simulink model "PressuredropFittingSimulation"  (R2022a)
settings: Solver=VariableStepAuto  StartTime=0.0  StopTime=10.0  RelTol=1e-3
settings Model: Creator=StephenDennis  LastModifiedBy=StephenDennis

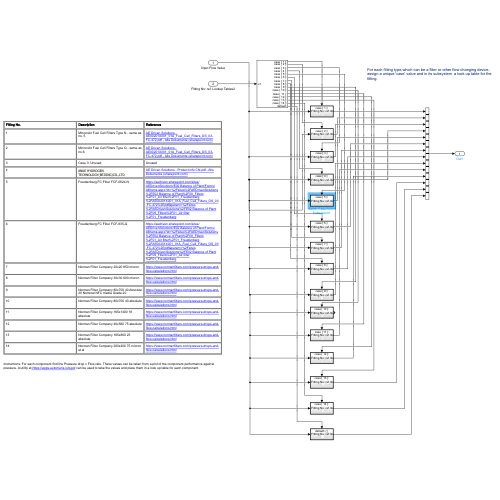
[thumbnail: Simulink's stored preview of the top-level diagram]
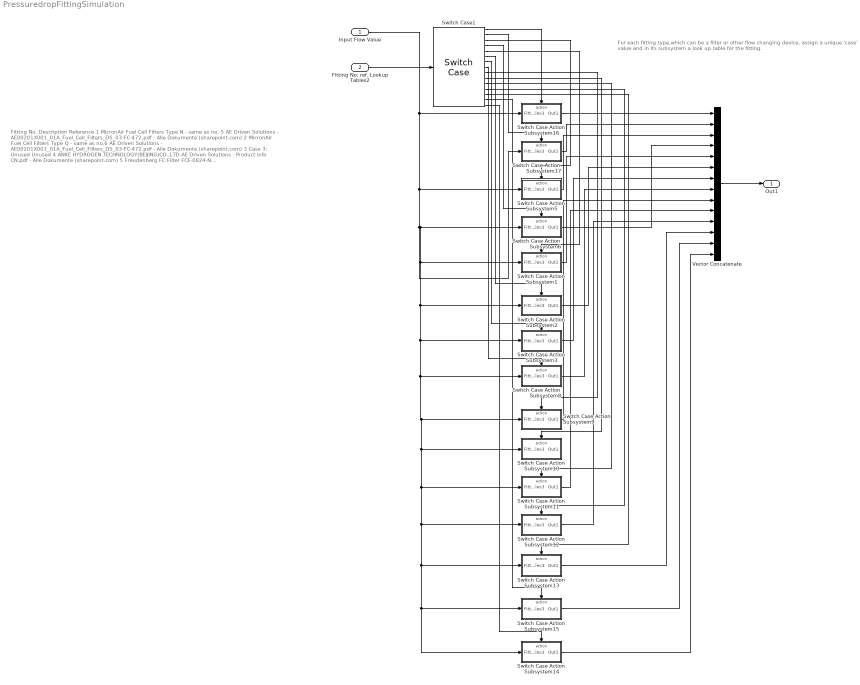
== system PressuredropFittingSimulation ==
  note: Fitting No.
      | Description
      | Reference
      |
      | 1
      | MicronAir Fuel Cell Filters Type N - same as no. 5
      | AE Driven Solutions - AE00201X001_01A_Fuel_Cell_Filters_DS_03-FC-472.pdf - Alle Dokumente (sharepoint.com)
      |
      | 2
      | MicronAir Fuel Cell Filters Type Q - same as no.6
      | AE Driven Solutions - AE00201X001_01A_Fuel_Cell_Filters_DS_03-FC-472.pdf - Alle Dokumente (sharepoint.com)
      |
      | 3
      | Case 3: Unused
      | Unused
      |
      | 4
      | ANKE HYDROGEN TECHNOLOGY(BEIJING)CO.,LTD
      | AE Driven Solutions - Product info CN.pdf - Alle Dokumente (sharepoint.com)
      |
      | 5
      | Freudenberg FC Filter FCF-0824-N
      | https://aedriven.sharepoint.com/sites/AEDrivenSolutions/E02 Balance of Plant/Forms/AllItems.aspx?id=%2Fsites%2FAEDrivenSolutions%2FE02 Balance of Plant%2F09_Filters%2F01_Air filter%2F01_Freudenberg%2FAE00201X001_01A_Fuel_Cell_Filters_DS_03-FC-472%2Epdf&parent=%2Fsites%2FAEDrivenSolutions%2FE02 Balance of Plant%2F09_Filters%2F01_Air filter%2F01_Freudenberg
      |
      | 6
      | Freudenberg FC Filter FCF-835-Q
      | https://aedriven.sharepoint.com/sites/AEDrivenSolutions/E02 Balance of Plant/Forms/AllItems.aspx?id=%2Fsites%2FAEDrivenSolutions%2FE02 Balance of Plant%2F09_Filters%2F01_Air filter%2F01_Freudenberg%2FAE00201X001_01A_Fuel_Cell_Filters_DS_03-FC-472%2Epdf&parent=%2Fsites%2FAEDrivenSolutions%2FE02 Balance of Plant%2F09_Filters%2F01_Air filter%2F01_Freudenberg
      |
      | 7
      | Norman Filter Company 20x20 850 micron
      | https://www.normanfilters.com/pressure-drops-and-flow-calculations.html
      |
      | 8
      | Norman Filter Company 30x30 600 micron
      | https://www.normanfilters.com/pressure-drops-and-flow-calculations.html
      |
      | 9
      | Norman Filter Company 80x700 40 Absolute 20 Nominal NFC media Grade 20
      | https://www.normanfilters.com/pressure-drops-and-flow-calculations.html
      |
      | 10
      | Norman Filter Company 80x700 40 absolute
      | https://www.normanfilters.com/pressure-drops-and-flow-calculations.html
      |
      | 11
      | Norman Filter Company 165x1400 18 absolute
      | https://www.normanfilters.com/pressure-drops-and-flow-calculations.html
      |
      | 12
      | Norman Filter Company 40x560 75 absolute
      | https://www.normanfilters.com/pressure-drops-and-flow-calculations.html
      |
      | 13
      | Norman Filter Company 165x800 25 absolute
      | https://www.normanfilters.com/pressure-drops-and-flow-calculations.html
      |
      | 14
      | Norman Filter Company 200x200 75 micron et al
      | https://www.normanfilters.com/pressure-drops-and-flow-calculations.html
      |
      | Instructions: For each component find the Pressure drop v Flow rate. These values can be taken from a plot of the component performance against
      | pressure. A utility at https://apps.automeris.io/wpd/ can be used to take the values and place them in a look up table for each component.
  note: For each fitting type,which can be a filter or other flow changing device, assign a unique 'case' value and in its subsystem a look up table for the fitting.
  Input Flow Value : Inport
  Fitting No: ref. Lookup Tables2 : Inport  Port=2
  Switch Case Action Subsystem1 : Subsystem  TreatAsAtomicUnit=on
  Switch Case Action Subsystem10 : Subsystem  TreatAsAtomicUnit=on
  Switch Case Action Subsystem11 : Subsystem  TreatAsAtomicUnit=on
  Switch Case Action Subsystem12 : Subsystem  TreatAsAtomicUnit=on
  Switch Case Action Subsystem13 : Subsystem  TreatAsAtomicUnit=on
  Switch Case Action Subsystem14 : Subsystem  TreatAsAtomicUnit=on
  Switch Case Action Subsystem15 : Subsystem  TreatAsAtomicUnit=on
  Switch Case Action Subsystem16 : Subsystem  TreatAsAtomicUnit=on
  Switch Case Action Subsystem17 : Subsystem  TreatAsAtomicUnit=on
  Switch Case Action Subsystem2 : Subsystem  TreatAsAtomicUnit=on
  Switch Case Action Subsystem3 : Subsystem  TreatAsAtomicUnit=on
  Switch Case Action Subsystem5 : Subsystem  TreatAsAtomicUnit=on
  Switch Case Action Subsystem6 : Subsystem  TreatAsAtomicUnit=on
  Switch Case Action Subsystem8 : Subsystem  TreatAsAtomicUnit=on
  Switch Case Action Subsystem9 : Subsystem  TreatAsAtomicUnit=on
  Switch Case1 : SwitchCase  CaseConditions={1,2,3,4,5,6,7,8,9,10,11,12,13,14}
  Vector Concatenate : Concatenate  NumInputs=14
  Out1 : Outport
  wires:
  Switch Case1/15 -> Switch Case Action Subsystem14/Action
  Switch Case Action Subsystem16/1(Out1) -> Vector Concatenate/1
  Switch Case1/2 -> Switch Case Action Subsystem17/Action
  Switch Case1/1 -> Switch Case Action Subsystem16/Action
  Vector Concatenate/1 -> Out1/1
  Switch Case Action Subsystem6/1(Out1) -> Vector Concatenate/4
  Fitting No: ref. Lookup Tables2/1 -> Switch Case1/1
  Switch Case Action Subsystem5/1(Out1) -> Vector Concatenate/3
  Switch Case1/3 -> Switch Case Action Subsystem5/Action
  Switch Case Action Subsystem17/1(Out1) -> Vector Concatenate/2
  Input Flow Value/1 -> Switch Case Action Subsystem17/1(Fitting No: ref. Lookup Tables3), Switch Case Action Subsystem15/1(Fitting No: ref. Lookup Tables3), Switch Case Action Subsystem14/1(Fitting No: ref. Lookup Tables3), Switch Case Action Subsystem13/1(Fitting No: ref. Lookup Tables3), Switch Case Action Subsystem12/1(Fitting No: ref. Lookup Tables3), Switch Case Action Subsystem11/1(Fitting No: ref. Lookup Tables3), Switch Case Action Subsystem10/1(Fitting No: ref. Lookup Tables3), Switch Case Action Subsystem9/1(Fitting No: ref. Lookup Tables3), Switch Case Action Subsystem8/1(Fitting No: ref. Lookup Tables3), Switch Case Action Subsystem3/1(Fitting No: ref. Lookup Tables3), Switch Case Action Subsystem2/1(Fitting No: ref. Lookup Tables3), Switch Case Action Subsystem1/1(Fitting No: ref. Lookup Tables3), Switch Case Action Subsystem6/1(Fitting No: ref. Lookup Tables3), Switch Case Action Subsystem5/1(Fitting No: ref. Lookup Tables3), Switch Case Action Subsystem16/1(Fitting No: ref. Lookup Tables3)
  Switch Case1/4 -> Switch Case Action Subsystem6/Action
  Switch Case1/5 -> Switch Case Action Subsystem1/Action
  Switch Case1/6 -> Switch Case Action Subsystem2/Action
  Switch Case Action Subsystem1/1(Out1) -> Vector Concatenate/5
  Switch Case Action Subsystem2/1(Out1) -> Vector Concatenate/6
  Switch Case1/7 -> Switch Case Action Subsystem3/Action
  Switch Case1/8 -> Switch Case Action Subsystem8/Action
  Switch Case1/9 -> Switch Case Action Subsystem9/Action
  Switch Case1/10 -> Switch Case Action Subsystem10/Action
  Switch Case1/11 -> Switch Case Action Subsystem11/Action
  Switch Case1/12 -> Switch Case Action Subsystem12/Action
  Switch Case1/13 -> Switch Case Action Subsystem13/Action
  Switch Case Action Subsystem3/1(Out1) -> Vector Concatenate/7
  Switch Case Action Subsystem8/1(Out1) -> Vector Concatenate/8
  Switch Case Action Subsystem9/1(Out1) -> Vector Concatenate/9
  Switch Case Action Subsystem11/1(Out1) -> Vector Concatenate/10
  Switch Case Action Subsystem12/1(Out1) -> Vector Concatenate/11
  Switch Case Action Subsystem13/1(Out1) -> Vector Concatenate/12
  Switch Case Action Subsystem14/1(Out1) -> Vector Concatenate/14
  Switch Case Action Subsystem15/1(Out1) -> Vector Concatenate/13
  Switch Case1/14 -> Switch Case Action Subsystem15/Action

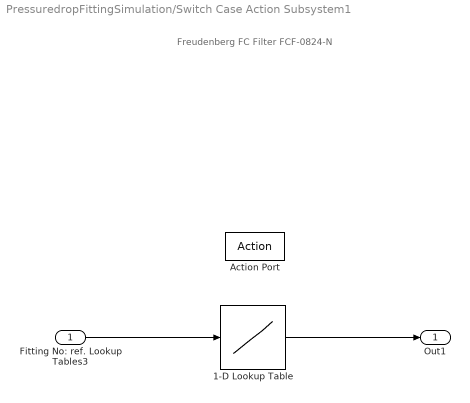
== system PressuredropFittingSimulation/Switch Case Action Subsystem1 ==
  note: Freudenberg FC Filter FCF-0824-N
  Fitting No: ref. Lookup Tables3 : Inport
  Action Port : ActionPort  ActionPortLabel=case [ 5 ]:
  1-D Lookup Table : Lookup_n-D  NumberOfTableDimensions=1  BreakpointsForDimension1=[0.225255973;4.325938567;10.54607509;16.30546075;21.37372014;28.05460751;33.29564846;38.70947099;44.00170648;50.70819113;55.99585568;61.59068747;66.98805461;72.05631399;77.12457338;82.19283276;87.26109215;92.32935154;97.39761092;102.4658703;107.5341297;112.6023891;117.6706485;122.7389078;127.8071672;132.8754266;137.943686;143.0119454;148.0802048;153.1484642;158.2167235;163.2849829;168.3532423;173.4215017;178.4897611;183.5580205;188.6262799;193.6945392;198.7627986;203.831058;208.8993174;213.9675768;219.0358362;224.1040956;229.1723549;234.2406143;239.3088737;244.3771331;249.4453925;254.5136519;259.5819113;264.6501706;269.71843;274.7866894;279.8549488;284.9232082;289.9914676;295.059727;300.1279863]  Table=[2.196382429;4.992617202;0.839793282;2.777777778;8.06319004;6.65374677;9.318475452;11.25645995;16.12833764;19.57364341;25.7567368;30.74012551;26.82640357;29.82147052;33.4331689;36.78059666;40.30420484;44.62062485;48.67277425;52.30209067;54.92717876;58.97932817;63.38383838;67.96452901;74.39511393;80.20906742;86.99201315;94.65586093;103.1125206;112.802443;123.0209067;133.9440921;145.3077284;157.3760864;170.0610759;182.7460653;196.2238666;209.7016678;223.3556495;237.5381724;252.0730561;265.815128;280.2619215;294.5325346;309.2435988;324.3070237;338.9299977;353.9053324;369.1449377;384.7369039;399.9765093;416.1851069;432.9222457;450.0117454;466.7488842;484.0145642;501.2802443;519.0744656;536.6925065]  InternalRulePriority=Speed  RndMeth=Simplest
  Out1 : Outport
  wires:
  Fitting No: ref. Lookup Tables3/1 -> 1-D Lookup Table/1
  1-D Lookup Table/1 -> Out1/1

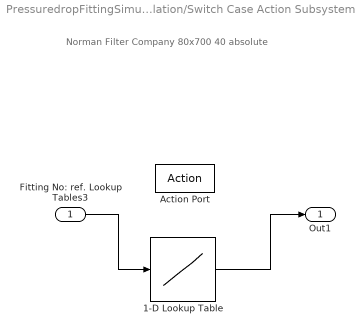
== system PressuredropFittingSimulation/Switch Case Action Subsystem10 ==
  note: Norman Filter Company 80x700 40 absolute
  Fitting No: ref. Lookup Tables3 : Inport
  Action Port : ActionPort  ActionPortLabel=case [ 10 ]:
  1-D Lookup Table : Lookup_n-D  NumberOfTableDimensions=1  BreakpointsForDimension1="[5.731513805\t36.87083466\t68.01015551\t99.14947636\t130.2887972\t161.4281181\t192.5674389\t223.7067598\t254.8460806\t285.9854015\t319.5511629\t347.1752557\t379.403364\t410.5426849\t441.6820057\t472.8213266\t505.9204648\t532.6021618\t566.2392891\t597.37861\t628.9897387\t661.4770821\t692.5844761\t723.2569555\t754.3490955\t782.9760394\t815.9498238\t847.3778166\t878.4817518\t908.0978072\t940.9019359\t969.2625566\t1001.088896\t1033.059497\t1064.021447\t1095.607744\t1126.747064\t1157.886385\t1188.08209\t1218.666343\t1252.578229\t1282.443669\t1313.58299\t1344.72231\t1375.861631\t1404.503146\t1438.140273\t1469.279594\t1500.418915\t1531.558235\t1562.697556\t1593.836877\t1624.302187\t1653.958683\t1684.423992\t1715.563313\t1746.702634\t1777.841955\t1808.981276\t1840.120597\t1871.259917\t1902.399238\t1933.538559\t1964.67788\t1991.975337]"  Table="[0.699801063\t0.441503285\t0.567587624\t0.66857184\t0.739494281\t0.924117777\t1.251420046\t1.487828181\t1.74174803\t2.153273303\t2.335270042\t2.787736162\t3.44914012\t4.070805958\t4.674960082\t5.121508782\t5.432678465\t5.614412019\t6.723830589\t7.389275711\t8.046613559\t8.717083537\t9.404423003\t10.15898256\t10.99651675\t11.97860858\t12.78445989\t13.65971572\t14.42213804\t14.9686396\t15.97143584\t16.60239751\t17.58855759\t18.48668233\t19.51709572\t20.69793494\t21.81114485\t22.93967751\t24.12755543\t25.37020037\t26.92709473\t28.21070335\t29.51970395\t30.63169777\t32.01074523\t33.25665216\t34.3310473\t35.67944926\t37.04536293\t38.73524331\t40.09677905\t41.53273958\t43.32623092\t45.24793303\t46.96137083\t48.55931471\t50.04343245\t51.74206869\t53.07733686\t54.66214695\t56.3170039\t58.31333927\t60.23087192\t62.32352171\t63.53620789]"  InternalRulePriority=Speed  RndMeth=Simplest
  Out1 : Outport
  wires:
  Fitting No: ref. Lookup Tables3/1 -> 1-D Lookup Table/1
  1-D Lookup Table/1 -> Out1/1

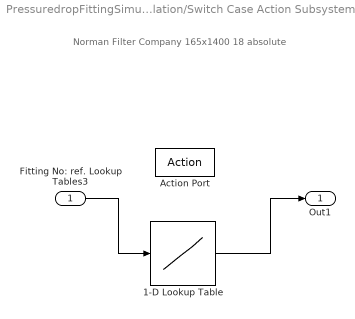
== system PressuredropFittingSimulation/Switch Case Action Subsystem11 ==
  note: Norman Filter Company 165x1400 18 absolute
  Fitting No: ref. Lookup Tables3 : Inport
  Action Port : ActionPort  ActionPortLabel=case [ 11 ]:
  1-D Lookup Table : Lookup_n-D  NumberOfTableDimensions=1  BreakpointsForDimension1=[19.50347696 50.62498646 81.74649596 112.8680055 143.989515 175.1110245 206.232534 237.3540435 268.475553 299.5970625 330.718572 361.8400815 392.961591 424.0831005 455.20461 486.3261195 517.447629 548.5691385 579.6906479 610.8121574 641.9336669 673.0551764 704.1766859 735.2981954 766.4197049 797.5412144 828.6627239 859.7842334 890.9057429 922.0272524 953.1487619 984.2702714 1015.391781 1046.51329 1077.6348 1108.756309 1139.877819 1170.999328 1202.120838 1233.242347 1264.363857 1295.485366 1326.606876 1357.728385 1388.849895 1419.971404 1451.092914 1482.214423 1513.335933 1544.457442 1575.578952 1606.700461 1637.821971 1668.94348 1700.06499 1731.186499 1762.308009 1793.429518 1824.551028 1855.672537 1886.794047 1917.915556 1949.037066 1980.158575 1998.548558]  Table=[0.0953884904119775 0.5159225300020438 1.0021650132780877 1.4066369888560644 1.7746042734973884 2.0023935449420236 2.3440774521089764 2.677000233451139 3.088773147216429 3.491784935156943 3.921080100571814 4.4423670871470335 5.071707958894706 5.529622802003914 5.8835722853255845 6.453045463937173 7.031279768373551 7.565708443685949 8.152703873947118 8.774743807507463 9.53696175426451 10.167762813649645 10.894936257107517 11.429364932419915 12.165299501702592 12.980084203408381 13.707257646866267 14.42566996449932 15.152843407957207 16.12532837450928 16.817457314667976 17.535869632301058 18.4207433406052 19.28809479725976 20.17880925611375 21.110408968816827 21.995282677120997 22.915200888724314 23.931491484400368 24.87769307347807 25.87646141750453 26.936557642304564 28.057981747878145 29.100555721028584 30.1518908200038 31.2557926739278 32.342172276202206 33.48111863342538 34.646348368122915 35.84662260611964 37.04689684411636 38.17708207551473 39.39487856516105 40.621436180632145 41.90056055105201 43.16216266982228 44.41500366276776 45.78173929143557 47.1046692909794 48.445121542172814 49.79433491919103 51.17859279950841 52.57161180565059 53.9295863084936 54.38516485138287]  InternalRulePriority=Speed  RndMeth=Simplest
  Out1 : Outport
  wires:
  Fitting No: ref. Lookup Tables3/1 -> 1-D Lookup Table/1
  1-D Lookup Table/1 -> Out1/1

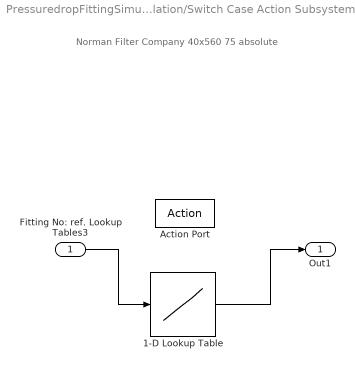
== system PressuredropFittingSimulation/Switch Case Action Subsystem12 ==
  note: Norman Filter Company 40x560 75 absolute
  Fitting No: ref. Lookup Tables3 : Inport
  Action Port : ActionPort  ActionPortLabel=case [ 12 ]:
  1-D Lookup Table : Lookup_n-D  NumberOfTableDimensions=1  BreakpointsForDimension1="[93.06340850501508 124.18491800437602 155.30642750373698 186.4279370030979 217.5494465024588 248.67095600181977 279.7924655011807 310.91397500054165 339.20625636359705 381.6446784081802 421.25387231645766 460.86306622473523 499.05764606486 538.6668399731376 576.8614198132624 615.0559996533872 656.0798076298175 694.2743874699423 731.0543532419143 772.0781612183447 808.8581269903167 848.4673208985943 888.0765148068717 924.8564805788437 964.4656744871213 1002.6602543272461 1040.8548341673709 1079.0494140074957 1117.2439938476205 1155.4385736877452 1192.2185394597172  1231.8277333679948 1268.6076991399668 1306.8022789800916 1343.5822447520636 1378.9475964558828 1415.727562227855 1453.9221420679798 1492.1167219081044 1527.4820736119239 1565.6766534520486 1602.4566192240206 1639.2365849959926 1677.4311648361174 1712.7965165399366 1749.5764823119086 1786.3564480838807 1823.1364138558527 1857.087151491519 1895.2817313316439 1930.6470830354633 1967.4270488074353 1994.3047161023378]"  Table="[0.039901360188252966 0.1450348700857944 0.19760162503455092 0.30273513493206394 0.31149626075686854 0.3377796382312539 0.504241028902328 0.7419595762817295 1.2090249285857055 1.7520756642336437 2.041192816451826  2.426682352742745 2.8379859204817137 3.2756771648120377 3.6795233456882244 4.143028621466598 4.670782153293445 5.219186910278722 5.684986766630274  6.254042748774012 6.763439636015576 7.396743874207772 8.08511804615587 8.71842228434808 9.406796456296135 10.102054369963696 10.811079767070211 11.531578067042503 12.339270428794919 13.121722404242547 13.94088766886074 14.840363253539564 15.643466454145639 16.593422811433967 17.551639658785675 18.390079400218426 19.353803240945723 20.324410823392498 21.36156124246091 22.320695922041878 23.401443372000358 24.461539596800378 25.54572891761859 26.712523139070555 27.770324783297426 28.926793392170183 30.099324065055043 31.30397886596417 32.460447474836926 33.72292570618967 34.95006739671577 36.202908389661246 37.23088048643703]"  InternalRulePriority=Speed  RndMeth=Simplest
  Out1 : Outport
  wires:
  Fitting No: ref. Lookup Tables3/1 -> 1-D Lookup Table/1
  1-D Lookup Table/1 -> Out1/1

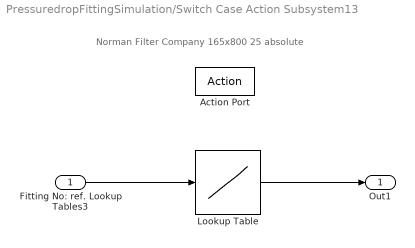
== system PressuredropFittingSimulation/Switch Case Action Subsystem13 ==
  note: Norman Filter Company 165x800 25 absolute
  Fitting No: ref. Lookup Tables3 : Inport
  Action Port : ActionPort  ActionPortLabel=case [ 13 ]:
  " Lookup Table" : Lookup_n-D  NumberOfTableDimensions=1  BreakpointsForDimension1="[11.015792552154437 42.13730205151538 73.25881155087632 104.38032105023723 135.5018305495982 166.6233400489591 197.74484954832008 228.866359047681 259.98786854704196 291.10937804640287 322.23088754576384 353.35239704512475 384.47390654448566 415.5954160438466 446.7169255432076 477.83843504256845 508.9599445419294 540.0814540412904  571.2029635406514 602.3244730400122 633.1630597257425 663.435800784212 695.6890015380951 726.810511037456 757.9320205368169 788.1104539907427 820.1750395355389 851.2965490348997 882.4180585342607 913.5395680336217 944.6610775329825 974.3679729641908 1006.9040965317045 1038.0256060310653 1069.1471155304264 1099.7027794025262 1129.9755204609955 1162.5116440285092 1193.63315352787  1224.7546630272311 1255.876172526592 1286.9976820259528 1318.119191525314 1349.2407010246748 1380.3622105240356 1411.4837200233967 1442.6052295227576 1473.7267390221184 1504.8482485214795 1535.9697580208403 1567.0912675202014 1598.2127770195623 1629.3342865189231 1660.4557960182842 1692.1431511449064 1722.698815017006 1752.2485311073083 1784.9418340157279 1816.063343515089 1847.1848530144498 1878.3063625138107 1909.4278720131717 1940.5493815125324 1971.6708910118937 1992.4185640114674]"  Table=[-0.07224105036908668 -0.15284340795720652 -0.222932414555558 -0.31930479862828065 -0.345588176102666 -0.24921579202991495 -0.03310802168498128 -0.2170916640056788 -0.24921579202992916 -0.17036565960677308 0.2676906316329024 0.99486407509076 1.0561919558643211 1.4329203663304355 2.2418643174863604 2.536822220254436 2.457972087831294 2.5280610944296456 2.4930165911304556 2.708540286420387 3.066870332654446 3.346350246465363 3.3603680477850304 3.8509910939734766 4.122585994542078 4.185860792165585 4.534358908307368 4.97241519954704 5.3929492391371525 5.734633146304091 6.1639283117189905 6.574825112901806 6.908624006826415 7.092607649147098 7.250307913993396 7.760205436996372 8.174606688509101 8.581999039362003 8.967488575652922 9.352978111943841 9.791034403183517 10.264135197722382 10.632102482363706 10.912458508757112 11.574799621111495 11.884943475309186 12.366805395672827 12.874950693510854 13.234156852327402 13.963082520950195 14.332802030756525 14.802398374965449 15.310543672803476 16.05523936791093 16.414445526727476 17.0036020346920 17.26038089803255 17.76365890374568 18.324370956532462 18.928888638443226 19.623937953876847 20.181729631388706 20.558458041854834 21.040319962218476 21.350853199786187]  InternalRulePriority=Speed  RndMeth=Simplest
  Out1 : Outport
  wires:
  Fitting No: ref. Lookup Tables3/1 -> " Lookup Table"/1
  " Lookup Table"/1 -> Out1/1

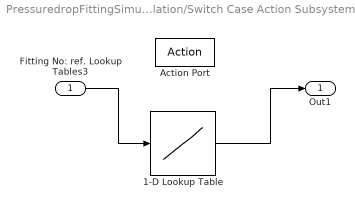
== system PressuredropFittingSimulation/Switch Case Action Subsystem14 ==
  Fitting No: ref. Lookup Tables3 : Inport
  Action Port : ActionPort  ActionPortLabel=default:
  1-D Lookup Table : Lookup_n-D  NumberOfTableDimensions=1  BreakpointsForDimension1=0  Table=0  InternalRulePriority=Speed  RndMeth=Simplest
  Out1 : Outport
  wires:
  Fitting No: ref. Lookup Tables3/1 -> 1-D Lookup Table/1
  1-D Lookup Table/1 -> Out1/1

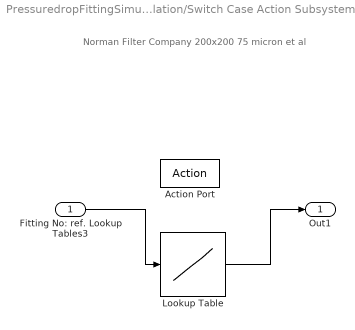
== system PressuredropFittingSimulation/Switch Case Action Subsystem15 ==
  note: Norman Filter Company 200x200 75 micron et al
  Fitting No: ref. Lookup Tables3 : Inport
  Action Port : ActionPort  ActionPortLabel=case [ 14 ]:
  " Lookup Table" : Lookup_n-D  NumberOfTableDimensions=1  BreakpointsForDimension1=|  Table=|  InternalRulePriority=Speed  RndMeth=Simplest
      BreakpointsForDimension1=|
      | [31.16364558	62.25757384	93.35150209	124.4454303	155.5393586	186.6332869	217.7272151	248.8211434	279.9150716	311.0089999	342.1029281	373.1968564	404.2907846	435.3847129	466.4786411	497.5725694	528.6664977	559.7604259	591.9415545	621.9482824	653.0422107	684.1361389	715.2300672	746.3239954	777.4179237	808.5118519	839.6057802	870.6997085	902.0291968	932.887565	963.9814932	995.7277416	1024.755989	1054.436557	1085.530485	1116.624414	1146.304982	1175.985549	1205.992277	1238.173406	1265.498373	1297.534542	1326.272869	1354.540077	1382.336164	1410.603372	1438.022563	1467.137787	1496.175918	1521.451207	1550.911511	1579.178718	1603.591307	1626.847509	1653.701356	1679.141843	1704.58233	1729.765842	1754.049943	1780.19711	1806.874287	1837.873085	1863.649616	1893.26594	1913.557757	1937.786792	1959.639518	1984.427684	2002.801369
      | ]
      Table=|
      | [-22.67333548	-21.7831509	-20.81586371	-19.69086666	-18.63946754	-17.44087255	-16.14765164	-15.0121406	-13.80303161	-12.43621276	-11.05887992	-9.702575063	-8.20958832	-6.895339426	-5.602118514	-3.804226027	-2.132501434	-0.45026285	1.230762582	2.987812257	4.75416277	6.383831399	8.339433753	10.04270032	12.09292859	14.08007292	16.14081519	18.42235127	20.33214961	22.64360189	24.55200811	26.82042417	29.17185582	31.30199043	33.37324669	35.75992268	38.06564094	40.45967672	42.72827251	45.29611265	47.63021869	50.3533424	52.80465996	55.56643232	58.09047166	60.74326845	63.02606621	65.57760158	67.96427758	70.57489741	73.33692705	75.93388287	78.19439097	80.79975797	83.41867635	85.98876307	88.57170023	91.06351614	93.84840954	96.02173913	99.13415431	102.2873634	105.1102083	107.6353185	110.0420212	112.7433659	115.3411305	118.3473232	119.4512922
      | ]
  Out1 : Outport
  wires:
  Fitting No: ref. Lookup Tables3/1 -> " Lookup Table"/1
  " Lookup Table"/1 -> Out1/1

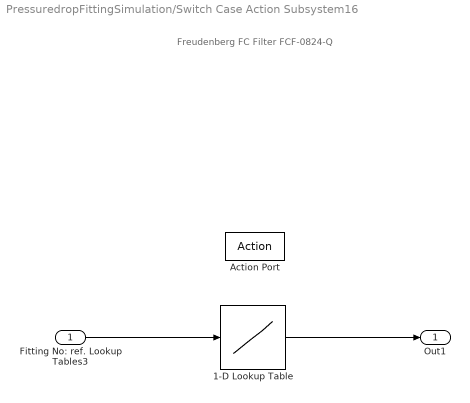
== system PressuredropFittingSimulation/Switch Case Action Subsystem16 ==
  note: Freudenberg FC Filter FCF-0824-Q
  Fitting No: ref. Lookup Tables3 : Inport
  Action Port : ActionPort  ActionPortLabel=case [ 1 ]:
  1-D Lookup Table : Lookup_n-D  NumberOfTableDimensions=1  BreakpointsForDimension1=[0.225255973;4.325938567;10.54607509;16.30546075;21.37372014;28.05460751;33.29564846;38.70947099;44.00170648;50.70819113;55.99585568;61.59068747;66.98805461;72.05631399;77.12457338;82.19283276;87.26109215;92.32935154;97.39761092;102.4658703;107.5341297;112.6023891;117.6706485;122.7389078;127.8071672;132.8754266;137.943686;143.0119454;148.0802048;153.1484642;158.2167235;163.2849829;168.3532423;173.4215017;178.4897611;183.5580205;188.6262799;193.6945392;198.7627986;203.831058;208.8993174;213.9675768;219.0358362;224.1040956;229.1723549;234.2406143;239.3088737;244.3771331;249.4453925;254.5136519;259.5819113;264.6501706;269.71843;274.7866894;279.8549488;284.9232082;289.9914676;295.059727;300.1279863]  Table=[2.196382429;4.992617202;0.839793282;2.777777778;8.06319004;6.65374677;9.318475452;11.25645995;16.12833764;19.57364341;25.7567368;30.74012551;26.82640357;29.82147052;33.4331689;36.78059666;40.30420484;44.62062485;48.67277425;52.30209067;54.92717876;58.97932817;63.38383838;67.96452901;74.39511393;80.20906742;86.99201315;94.65586093;103.1125206;112.802443;123.0209067;133.9440921;145.3077284;157.3760864;170.0610759;182.7460653;196.2238666;209.7016678;223.3556495;237.5381724;252.0730561;265.815128;280.2619215;294.5325346;309.2435988;324.3070237;338.9299977;353.9053324;369.1449377;384.7369039;399.9765093;416.1851069;432.9222457;450.0117454;466.7488842;484.0145642;501.2802443;519.0744656;536.6925065]  InternalRulePriority=Speed  RndMeth=Simplest
  Out1 : Outport
  wires:
  Fitting No: ref. Lookup Tables3/1 -> 1-D Lookup Table/1
  1-D Lookup Table/1 -> Out1/1

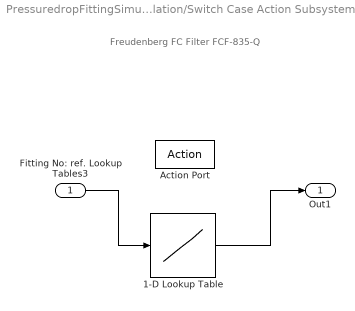
== system PressuredropFittingSimulation/Switch Case Action Subsystem17 ==
  note: Freudenberg FC Filter FCF-835-Q
  Fitting No: ref. Lookup Tables3 : Inport
  Action Port : ActionPort  ActionPortLabel=case [ 2 ]:
  1-D Lookup Table : Lookup_n-D  NumberOfTableDimensions=1  BreakpointsForDimension1=|  Table="[0.743908154\t3.467666354\t7.070056232\t7.860824742\t7.860824742\t7.94868791\t11.19962512\t12.78116214\t17.87722587\t19.45876289\t19.02920962\t22.00679475\t26.31208997\t32.11105904\t35.97703843\t38.61293346\t42.12746017\t46.60848172\t50.91377694\t56.09770384\t60.8423149\t65.58692596\t71.38589503\t78.15135895\t86.76194939\t96.33903468\t105.6525305\t114.7024367\t124.5431115\t134.4716495\t144.5759138\t154.9437676\t166.7174321\t177.7881912\t190.0011715\t203.7078257\t217.0630272\t229.8910497\t242.5433458\t255.8106842\t269.868791\t283.8390347\t297.8971415\t311.6916589\t325.1347235\t340.071462\t355.5353796\t370.3842549\t385.8481724\t401.3999531\t416.0731022\t432.239925\t448.6703374\t465.7377577\t482.0583411\t498.6644799\t517.3109966\t532.9311153\t550.5037488\t566.0806333]"  InternalRulePriority=Speed  RndMeth=Simplest
      | [1.454081633	6.505102041	11.55612245	16.60714286	21.65816327	26.70918367	31.76020408	36.81122449	41.8622449	46.91326531	51.50510204	57.4744898	62.5255102	67.57653061	72.62755102	77.67857143	82.72959184	87.78061224	92.83163265	97.88265306	102.9336735	107.9846939	113.0357143	118.0867347	123.1377551	128.1887755	133.2397959	138.2908163	143.3418367	148.3928571	153.4438776	158.494898	163.5459184	168.5969388	173.6479592	178.6989796	183.75	188.8010204	193.8520408	198.9030612	203.9540816	209.005102	214.0561224	219.1071429	224.1581633	229.2091837	234.2602041	239.3112245	244.3622449	249.4132653	254.4642857	259.5153061	264.5663265	269.3877551	274.6683673	279.7193878	285.0255102	289.8214286	294.872449	299.005102
      | ]
  Out1 : Outport
  wires:
  Fitting No: ref. Lookup Tables3/1 -> 1-D Lookup Table/1
  1-D Lookup Table/1 -> Out1/1

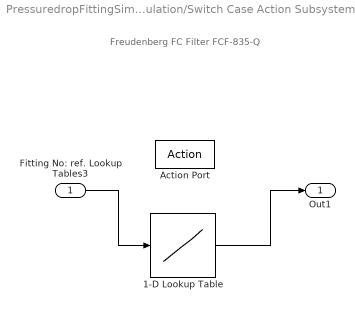
== system PressuredropFittingSimulation/Switch Case Action Subsystem2 ==
  note: Freudenberg FC Filter FCF-835-Q
  Fitting No: ref. Lookup Tables3 : Inport
  Action Port : ActionPort  ActionPortLabel=case [ 6 ]:
  1-D Lookup Table : Lookup_n-D  NumberOfTableDimensions=1  BreakpointsForDimension1=|  Table=|  InternalRulePriority=Speed  RndMeth=Simplest
      BreakpointsForDimension1=|
      | [1.454081633	6.505102041	11.55612245	16.60714286	21.65816327	26.70918367	31.76020408	36.81122449	41.8622449	46.91326531	51.50510204	57.4744898	62.5255102	67.57653061	72.62755102	77.67857143	82.72959184	87.78061224	92.83163265	97.88265306	102.9336735	107.9846939	113.0357143	118.0867347	123.1377551	128.1887755	133.2397959	138.2908163	143.3418367	148.3928571	153.4438776	158.494898	163.5459184	168.5969388	173.6479592	178.6989796	183.75	188.8010204	193.8520408	198.9030612	203.9540816	209.005102	214.0561224	219.1071429	224.1581633	229.2091837	234.2602041	239.3112245	244.3622449	249.4132653	254.4642857	259.5153061	264.5663265	269.3877551	274.6683673	279.7193878	285.0255102	289.8214286	294.872449	299.005102
      | ]
      Table=|
      | [0.743908154	3.467666354	7.070056232	7.860824742	7.860824742	7.94868791	11.19962512	12.78116214	17.87722587	19.45876289	19.02920962	22.00679475	26.31208997	32.11105904	35.97703843	38.61293346	42.12746017	46.60848172	50.91377694	56.09770384	60.8423149	65.58692596	71.38589503	78.15135895	86.76194939	96.33903468	105.6525305	114.7024367	124.5431115	134.4716495	144.5759138	154.9437676	166.7174321	177.7881912	190.0011715	203.7078257	217.0630272	229.8910497	242.5433458	255.8106842	269.868791	283.8390347	297.8971415	311.6916589	325.1347235	340.071462	355.5353796	370.3842549	385.8481724	401.3999531	416.0731022	432.239925	448.6703374	465.7377577	482.0583411	498.6644799	517.3109966	532.9311153	550.5037488	566.0806333
      | ]
  Out1 : Outport
  wires:
  Fitting No: ref. Lookup Tables3/1 -> 1-D Lookup Table/1
  1-D Lookup Table/1 -> Out1/1

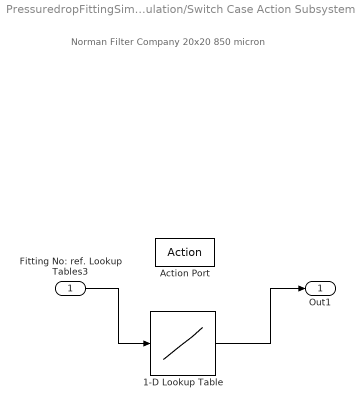
== system PressuredropFittingSimulation/Switch Case Action Subsystem3 ==
  note: Norman Filter Company 20x20 850 micron
  Fitting No: ref. Lookup Tables3 : Inport
  Action Port : ActionPort  ActionPortLabel=case [ 7 ]:
  1-D Lookup Table : Lookup_n-D  NumberOfTableDimensions=1  BreakpointsForDimension1="[32.38865968475616 62.3484608060933 93.48778165661693  124.62710250714059 155.76642335766422 187.84935999153703 218.0450650587115 249.18438590923512 280.3237067597588 311.46302761028244 342.60234846080607  373.7416693113297 404.4091822701788  436.02031101237696 467.1596318629006  498.2989527134242 529.4382735639479  560.5775944144716  594.1433558507503  620.9690045488204 654.2314609118797 685.1348778165661 716.2741986670898 747.4135195176134  779.8593852989283 807.2657206329056 840.8314820691843  871.9708029197079 903.1101237702317 934.7212525124298  966.5682852004654  995.5844705384534 1027.6674071723262  1058.8067280228497  1089.9460488733735 1121.085369723897 1149.393843224373 1178.57334667871 1207.7528501330469 1239.9809584258965 1267.3458161430233  1300.1836454035754 1329.2615286966288 1354.5213973585917 1388.6004443033955  1412.6626467788003 1439.5556966042525  1467.992844984276 1496.0439687256571  1523.9367233845176  1552.5873872240104  1576.8517930815613  1601.1970802919705  1628.3217449006086 1654.7000952078704  1681.0784455151322  1704.2399238337034  1729.9748997432273 1754.937826375465  1781.7343700412566 1806.7570385818558  1833.7511900983814  1852.1516978736906 1876.9216121866073 1902.616995825501  1925.6992896028123  1950.9280500521372 1972.51714962283  1988.7400825134878  2005.7251666137731]"  Table=[1.059103903582752 1.925621024526862 2.7311598565557773 3.6680365416328726 4.499842944271393 5.418478260869563 6.504934167473749 7.520613564379772 8.5625605318954 9.694011814080923 10.856595031803778 11.93356542679895 13.009660236107095 14.402717064104905 15.646048739627773 16.933159699500052 18.229026516242172 19.621207758552984 20.79186582205587 21.93479700547077 23.910847970054704 25.38256157893359 27.019906813601025 28.553932937203896 29.933586568916255 31.24029931581039 33.36790304426354 35.010112643858676 36.87024579221527 38.63892887993089 40.40469334868989 41.85583069392456 44.190142135434385 46.0463837918488 48.025207444441534 50.02154281077401 51.86610999136194 53.5528472391415 55.782896631154614 57.787987854356984 59.71573567520875 61.69018139936654 63.987733209299584 65.90332011783207 68.15242071490272 70.18297341395527 72.24838276226124 74.35406905216868 76.47298641467947 78.58718908502956 80.59762041874049 82.92605292778053 84.6483299740858 87.18139936654188 89.37255254822918 91.25287281103577 93.54885305691523 95.61037091327906 97.53957804360914 99.75645155485171 101.96566369133313 104.36951122948459 106.28335912755541 108.42408100585467 110.57839597776251 112.69731334027331 114.9405927357986 117.10660891081275 118.95219230076135 119.59120357040021]  InternalRulePriority=Speed  RndMeth=Simplest
  Out1 : Outport
  wires:
  Fitting No: ref. Lookup Tables3/1 -> 1-D Lookup Table/1
  1-D Lookup Table/1 -> Out1/1

== system PressuredropFittingSimulation/Switch Case Action Subsystem5 ==
  Fitting No: ref. Lookup Tables3 : Inport
  Action Port : ActionPort  ActionPortLabel=case [ 3 ]:
  1-D Lookup Table1 : Lookup_n-D  NumberOfTableDimensions=1  BreakpointsForDimension1=[ 0 100]  Table=[0 0]  InternalRulePriority=Speed  RndMeth=Simplest
  Out1 : Outport
  wires:
  Fitting No: ref. Lookup Tables3/1 -> 1-D Lookup Table1/1
  1-D Lookup Table1/1 -> Out1/1

== system PressuredropFittingSimulation/Switch Case Action Subsystem6 ==
  note: ANKE HYDROGEN TECHNOLOGY(BEIJING)CO.,LTD
  Fitting No: ref. Lookup Tables3 : Inport
  Action Port : ActionPort  ActionPortLabel=case [ 4 ]:
  1-D Lookup Table1 : Lookup_n-D  NumberOfTableDimensions=1  BreakpointsForDimension1=|  Table=|  InternalRulePriority=Speed  RndMeth=Simplest
      BreakpointsForDimension1=|
      | [40.54653548	42.28265535	43.96771288	45.65277041	47.44388051	48.87991089	50.707943	52.39300053	54.07805806	55.76311559	57.44817312	59.13323065	60.5826158	62.35015866	64.03521619	65.72027372	67.40533125	69.09038878	70.7754463	72.46050383	74.14556136	75.83061889	77.65928928	79.22945652	80.88579148	82.57084901	84.25590654	85.94096407	87.6260216	89.31107913	90.99613666	92.68119419	94.36625171	96.05130924	97.73636677	99.56439888	101.1064818	102.8451548	104.5036299	105.8552803	107.1889087	108.5283943	110.047768	111.3700141	112.5955104	113.8210068	115.0465032	116.2990326	117.650683	119.0616164	120.5047996	120.6378305	122.0505555	123.5962553	125.3422853	126.8036092	128.4302137	130.212021	131.9396305	133.4385232	135.2671936	136.7023143	138.2318135	139.709618
      | ]
      Table=|
      | [1.513496985	1.577270378	1.641400047	1.724341085	1.78535745	1.868479472	1.935712474	1.979149636	2.04926474	2.127075405	2.225407564	2.323739723	2.431503876	2.536650223	2.669184872	2.811125206	2.961616162	3.110396993	3.260887949	3.410523843	3.555884426	3.69440451	3.834104759	3.932325581	4.030443975	4.091153394	4.149297627	4.197523138	4.210862109	4.238224101	4.263875969	4.298933521	4.348527132	4.420352361	4.515264271	4.645119724	4.811970872	4.971183463	5.190612555	5.387855297	5.602249582	5.875720327	6.057391541	6.296679587	6.504192506	6.711705426	6.918042636	7.130949992	7.342670112	7.54745002	7.83604896	7.729870801	7.972850991	8.194276486	8.407327621	8.632816537	8.813257174	9.079586563	9.262474878	9.459341085	9.706347193	9.877680916	10.05999088	10.24589147
      | ]
  Out1 : Outport
  wires:
  Fitting No: ref. Lookup Tables3/1 -> 1-D Lookup Table1/1
  1-D Lookup Table1/1 -> Out1/1

== system PressuredropFittingSimulation/Switch Case Action Subsystem8 ==
  note: Norman Filter Company 30x30 600 micron
  Fitting No: ref. Lookup Tables3 : Inport
  Action Port : ActionPort  ActionPortLabel=case [ 8 ]:
  1-D Lookup Table : Lookup_n-D  NumberOfTableDimensions=1  BreakpointsForDimension1=[31.209139955569668 63.242412600845171 90.989975171280804 113.30371310695017 207.28784512853059 242.57907542579073 279.6159949222469 324.20184068549662 356.75658521104407 393.84068549666767 432.56038647342984 466.45192002538874 491.50491907331002 526.60742621390034 569.54194435628892 602.2682553878999 635.24119327197707 662.48809901618529 693.39151592087171 722.99746112345281 754.2075531577276 791.67767808199403 791.67767808199403 829.2250079339891 829.2250079339891 829.2250079339891 859.07472054726895 881.87876864487453 913.3719454141542 932.83402094573148 966.19757899986394 999.35893367185008 1018.2312493388342 1050.314185972707 1082.0196762932401 1115.7382136182516 1149.3938432243731 1187.6102824500158 1216.3905638421666 1255.5506188511583 1287.7009566124132 1328.79879403364 1356.5175076695227 1393.6555288570521 1417.919934714603 1448.4020945731513 1462.2024754046333 1492.2802284988891 1527.3119644557282 1558.4512853062517 1587.4674706442397 1619.3145033322753 1648.0947847244258 1671.2133714164816 1702.3526922670051 1722.357346874008 1748.401142494446 1777.3701470432666 1804.0916303626552 1836.1102295567543 1869.2378836650496 1899.2853062519832]  Table=[1.1129941178890448 0.76510351606054883 1.4558950559780612 2.5210192916786696 3.2144831557731095 3.6928448027641849 4.375071983875614 5.4024258566081329 5.4930072806548509 5.9690757270371364 6.6910771987074895 7.5735135329686045 8.2420961704578275 8.8536927728188886 9.8890728476821153 10.58954139727247 11.241487906708883 11.940861974190511 13.195868125539874 14.339601929167884 14.881370572991671 15.806989727807462 17.176864382378341 17.537151678024145 19.64058738842499 19.656960840771674 21.195316249160186 21.774731602978079 23.078798349169773 24.255974661675793 24.609127555427577 25.967803052116324 26.902837764340802 28.606176216527501 30.133161171897498 31.045249864030453 32.725223150014401 34.249742914729964 36.062517995968904 37.295877723389964 39.178977623298096 40.432211755995226 40.8011877339476 42.166444716383523 43.611161099913616 45.321544773970629 46.711281672905272 48.029585372876468 49.811402245896915 51.523658700451094 52.427944140512523 53.59263524970406 55.288482579902094 56.091102792974368 57.757342355312403 59.325224458812144 61.406588924080992 63.309181029163746 64.75940109415491 66.682479124676064 68.544558019003745 69.979642959976957]  InternalRulePriority=Speed  RndMeth=Simplest
  Out1 : Outport
  wires:
  Fitting No: ref. Lookup Tables3/1 -> 1-D Lookup Table/1
  1-D Lookup Table/1 -> Out1/1

== system PressuredropFittingSimulation/Switch Case Action Subsystem9 ==
  note: Norman Filter Company 80x700 40 Absolute 20 Nominal NFC media Grade 20
  Fitting No: ref. Lookup Tables3 : Inport
  Action Port : ActionPort  ActionPortLabel=case [ 9 ]:
  1-D Lookup Table : Lookup_n-D  NumberOfTableDimensions=1  BreakpointsForDimension1="[31.20913996\t62.34846081\t93.48778166\t124.6271025\t155.7664234\t186.9057442\t218.0450651\t249.1843859\t280.3237068\t311.4630276\t342.6023485\t373.7416693\t404.8809902\t436.020311\t467.1596319\t498.2989527\t529.4382736\t560.5775944\t591.7169153\t622.8562361\t653.995557\t685.1348778\t716.2741987\t747.4135195\t778.5528404\t809.6921612\t840.8314821\t871.2630911\t902.4024119\t934.2494446\t965.3887655\t996.5280863\t1030.812793\t1057.10822\t1089.075019\t1118.254522\t1149.393843\t1180.533164\t1211.672485\t1242.811806\t1274.658838\t1305.326351\t1336.229768\t1366.560276\t1398.50841\t1429.647731\t1460.787052\t1491.690469\t1523.065693\t1554.205014\t1586.523855\t1615.304136\t1647.622977\t1678.762298\t1709.547763\t1741.258697\t1770.655958\t1803.101824\t1835.166614\t1864.418703\t1896.50164 1927.876864\t1959.016185\t1988.740083]"  Table="[0.051867654\t0.218228935\t0.603486637\t0.796115488\t1.137593906\t1.426537183\t1.671701175\t1.829306599\t2.170785017\t2.556042719\t3.063882418\t3.495108368\t3.921956391\t4.412284376\t5.025194356\t5.655616051\t6.286037746\t6.898947727\t7.406787425\t8.186058686\t8.816480381\t9.534460644\t10.32248776\t11.0054446\t11.76720415\t12.55523126\t13.27321153\t14.06804876\t15.02182911\t16.29898549\t16.85143837\t17.27463812\t18.49316153\t20.26213648\t21.07301222\t22.31801167\t23.40373793\t24.47195246\t25.59270214\t26.8798131\t28.11256479\t29.50001485\t30.78492527\t32.05785263\t33.52364611\t34.74257257\t36.14350967\t37.65973222\t39.15990236\t40.43387954\t41.85743593\t43.2459689\t45.10950711\t46.59800277\t47.94437386\t49.82733117\t51.31538905\t53.11572792\t55.06856464\t56.62564785\t58.57958217\t60.3972332\t62.17467215\t63.88293982]"  InternalRulePriority=Speed  RndMeth=Simplest
  Out1 : Outport
  wires:
  Fitting No: ref. Lookup Tables3/1 -> 1-D Lookup Table/1
  1-D Lookup Table/1 -> Out1/1
